simulink model "LFC_oneArea"  (R2021b)
settings: Solver=FixedStepAuto  StartTime=0.0  StopTime=32  FixedStep=0.01  RelTol=1e-3
undefined symbols (not defined in the file or in its folder): sigbuilder_block
libraries: deeplib x1
settings Model: Creator=abc19  LastModifiedBy=abc19
settings SolverCC: AlgebraicLoopSolver=TrustRegion
settings DebuggingCC: SFMachineParentedDataDiag=warning
settings SFSimCC: SimTargetLang=C++

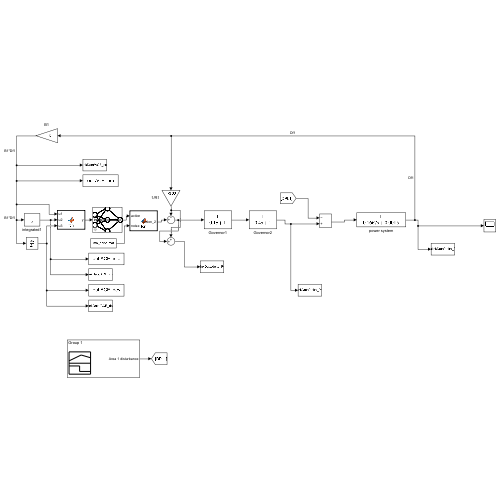
[thumbnail: Simulink's stored preview of the top-level diagram]
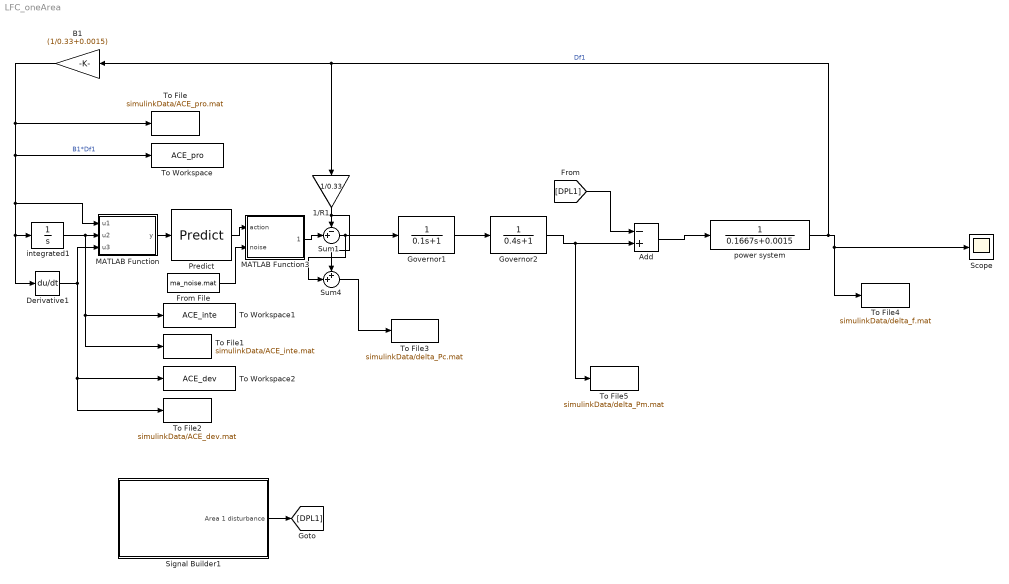
== system LFC_oneArea ==
  1/R1 : Gain  Gain=1/0.33
  Add : Sum  Inputs=-+
  B1 : Gain  Gain=(1/0.33+0.0015)
  Derivative1 : Derivative
  From File : FromFile  FileName=ma_noise.mat  SampleTime=0
  Governor1 : TransferFcn  Denominator=[0.1 1]
  Governor2 : TransferFcn  Denominator=[0.4 1]
  MATLAB Function : MATLAB Function  TreatAsAtomicUnit=on  SystemSampleTime=0.01
  MATLAB Function3 : MATLAB Function  TreatAsAtomicUnit=on  SystemSampleTime=0.01
  Predict : deeplib/Predict  Network=Network from MAT-file  NetworkFunction=squeezenet  NetworkFilePath=bbb.mat  MiniBatchSize=1  InputDataFormats={ '', '' }  Predictions=on  Activations={}  ForceInterpretedSim=off  EnableDLNetwork=on
      settings: SourceProductBaseCode=NN
  Scope : Scope
  Signal Builder1 : Subsystem  Tag=STV Subsys  LoadFcn=sigbuilder_block('load');  StartFcn=sigbuilder_block('start');  StopFcn=sigbuilder_block('stop');  ClipboardFcn=sigbuilder_block('clipboard');  mask(Sigbuilder block){tuvar=[0:10]}
      mask help: Simulink:masks:SigbuilderBlock_MD
      mask init:
      | if ~strcmp(get_param(bdroot(gcbh),'SimulationStatus'),'stopped') tuvar = sigbuilder_block('maskInit'); end
      settings: CopyFcn=sigbuilder_block('copy');  DeleteFcn=sigbuilder_block('delete');  ModelCloseFcn=sigbuilder_block('modelClose');  PreSaveFcn=sigbuilder_block('preSave');  PauseFcn=sigbuilder_block('pause');  ContinueFcn=sigbuilder_block('continue');  NameChangeFcn=sigbuilder_block('namechange');  OpenFcn=sigbuilder_block('open',[99.6 64.8 1141.8 523.2 ]);  CloseFcn=sigbuilder_block('close');
      mask Display: plot(0, 0, 100, 100,[2, 2, 32, 32, 2], [68, 8, 8, 68, 68],[32, 2], [38, 38], [32, 19, 2],[53, 60, 44], [32, 17, 17, 2],[16, 16, 31, 31]);txt = getActiveGroup(gcbh);text(2, 100, txt,'verticalAlignment', 'top');
  Sum1 : Sum  Inputs=-+|
  Sum4 : Sum  Inputs=++|
  To File : ToFile  Filename=simulinkData/ACE_pro.mat  SampleTime=0.01
  To File1 : ToFile  Filename=simulinkData/ACE_inte.mat  SampleTime=0.01
  To File2 : ToFile  Filename=simulinkData/ACE_dev.mat  SampleTime=0.01
  To File3 : ToFile  Filename=simulinkData/delta_Pc.mat  SampleTime=0.01
  To File4 : ToFile  Filename=simulinkData/delta_f.mat  SampleTime=0.01
  To File5 : ToFile  Filename=simulinkData/delta_Pm.mat  SampleTime=0.01
  To Workspace : ToWorkspace  VariableName=ACE_pro  SaveFormat=Timeseries  SampleTime=0.01
  To Workspace1 : ToWorkspace  VariableName=ACE_inte  SaveFormat=Timeseries  SampleTime=0.01
  To Workspace2 : ToWorkspace  VariableName=ACE_dev  SaveFormat=Timeseries  SampleTime=0.01
  integrated1 : TransferFcn  Denominator=[1 0]
  power system : TransferFcn  Denominator=[0.1667 0.0015]
  wires:
  [DPL1] -> Add/1
  power system/1 -> Scope/1, To File4/1, B1/1, 1/R1/1  "Df1"
  Governor2/1 -> To File5/1, Add/2
  Add/1 -> power system/1
  B1/1 -> Derivative1/1, integrated1/1, MATLAB Function/1(u1), To Workspace/1, To File/1  "B1*Df1"
  1/R1/1 -> Sum4/1, Sum1/1
  Governor1/1 -> Governor2/1
  Derivative1/1 -> To File2/1, To Workspace2/1, MATLAB Function/3(u3)
  integrated1/1 -> To File1/1, To Workspace1/1, MATLAB Function/2(u2)
  Sum1/1 -> Governor1/1, Sum4/2
  MATLAB Function/1(y) -> Predict/1
  MATLAB Function3/1(action_2) -> Sum1/2
  Predict/1 -> MATLAB Function3/1(action)
  Sum4/1 -> To File3/1
  From File/1 -> MATLAB Function3/2(noise)
  Signal Builder1/1(Area 1 disturbance) -> [DPL1]

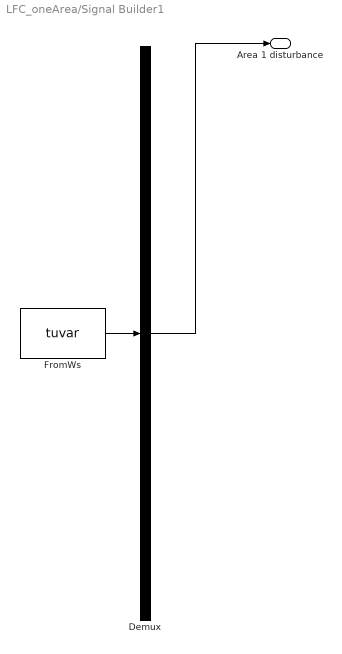
== system LFC_oneArea/Signal Builder1 ==
  Demux : Demux  Tag=STV Demux  Outputs=1
      settings: DisplayOption=none
  FromWs : FromWorkspace  Tag=STV FromWs  VariableName=tuvar
      SigBuilderData=|
      | common.afterFinalStr = 'Extrapolate'
      | common.sampleTime = 0
      | dataSet.timeRange = [0 200]
      | dataSet.name = 'Group 1'
      | sbobj.Groups.Name = 'Group 1'
      | sbobj.Groups.Signals.Name = 'Area 1 disturbance'
      | sbobj.Groups.Signals.XData = [0 4 4 8 8 12 12 16 16 20 20 24 24 28 28 200]
      | sbobj.Groups.Signals.YData = [0.01 0.01 -0.01 -0.01 0 0 0.01 0.01 0 0 0.02 0.02 -0.01 -0.01 0.02 0.02]
      | sbobj.Groups.TimeRange = [0 200]
  Area 1 disturbance : Outport  Tag=STV Outport
  wires:
  Demux/1 -> Area 1 disturbance/1
  FromWs/1 -> Demux/1

== matlab function LFC_oneArea/MATLAB Function ==
  settings: updateMethod=DISCRETE  sampleTime=0.01
  data: u1 input; y output; u2 input; u3 input
function y = fcn(u1, u2 ,u3)
num =1;
% net = coder.loadDeepLearningNetwork('bbb.mat');
statemax = [[0.0632, 0.0095, 0.5454]
                     [0.0305, 0.0970, 0.0190]
                     [0.0363, 0.0766, 0.0296]];
statemin = [[-0.0632, -0.0129, -0.5452]
                     [-0.0301, -0.1188, -0.0190]
                     [-0.0366, -0.0952, -0.0298]];

y1 = (u1-statemin(num ,1))/(statemax(num, 1) - statemin(num, 1));
y2 = (u2-statemin(num ,2))/(statemax(num, 2) - statemin(num, 2));
y3 = (u3-statemin(num ,3))/(statemax(num, 3) - statemin(num, 3));
y =[y1, y2,y3];
% action = predict(net, [u1, u2, u3]);
% action = action*(actionmax(num)-actionmin(num)) + actionmin(num);
% y = double(action);

== matlab function LFC_oneArea/MATLAB Function3 ==
  settings: updateMethod=DISCRETE  sampleTime=0.01
  data: action input; action_2 output; noise input
function action_2= fcn(action, noise)
num =1;
noise =1 ;

actionmax = [0.1058, 0.1458, 0.0943];
actionmin = [-0.0959, -0.1192 -0.0760];

action_2 = double(noise * ((action+1)*(actionmax(num)-actionmin(num))/2 + actionmin(num)));
